simulink model "lab7_t30"  (R2021a)
settings: Solver=VariableStepAuto  StartTime=0.0  StopTime=10.0  RelTol=1e-3
libraries: simulink x2
settings Model: Creator=reemb  LastModifiedBy=reemb

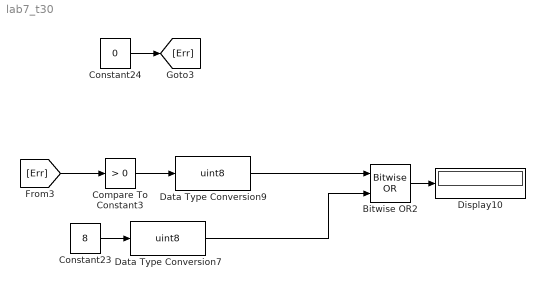
== system lab7_t30 ==
  Bitwise OR2 : simulink/Logic and Bit Operations/Bitwise Operator  logicop=OR  UseBitMask=off  NumInputPorts=2  BitMask=bin2dec('11011001')  BitMaskRealWorld=Stored Integer
  Compare To Constant3 : simulink/Logic and Bit Operations/Compare To Constant  relop=>  const=0  OutDataTypeStr=boolean
  Constant23 : Constant  Value=8
  Constant24 : Constant  Value=0
  Data Type Conversion7 : DataTypeConversion  OutDataTypeStr=uint8
  Data Type Conversion9 : DataTypeConversion  OutDataTypeStr=uint8
  Display10 : Display
  wires:
  [Err] -> Compare To Constant3/1
  Data Type Conversion9/1 -> Bitwise OR2/1
  Compare To Constant3/1 -> Data Type Conversion9/1
  Constant24/1 -> [Err]
  Constant23/1 -> Data Type Conversion7/1
  Data Type Conversion7/1 -> Bitwise OR2/2
  Bitwise OR2/1 -> Display10/1
